simulink model "torqueBalancing2012b"  (Simulink 8.1)
settings: Solver=FixedStepDiscrete  StartTime=0.0  StopTime="CONFIG.SIMULATION_TIME "  FixedStep=CONFIG.Ts  RelTol=1e-3
InitFcn:
  | cd(fileparts(which(bdroot)));
  | initTorqueBalancing;
values from neighbouring files (symbols this model uses):
  WBT_modelName = 'matlabTorqueBalancing'    [InitMeasure.m]    (also in initTorqueBalancing.m)
undefined symbols (not defined in the file or in its folder): bVectorConstraintsFeet, bVectorConstraintsLegs, CONFIG, ConstraintsMatrixFeet, ConstraintsMatrixLegs, DiscIntNeverNeededParam, gain, references, reg, ROBOT_DOF, ROBOT_DOF_FOR_SIMULINK, sat, SM, sm, WBT_robotName
libraries: WBToolboxLibrary x182, simulink x13
(part 2 of 4)

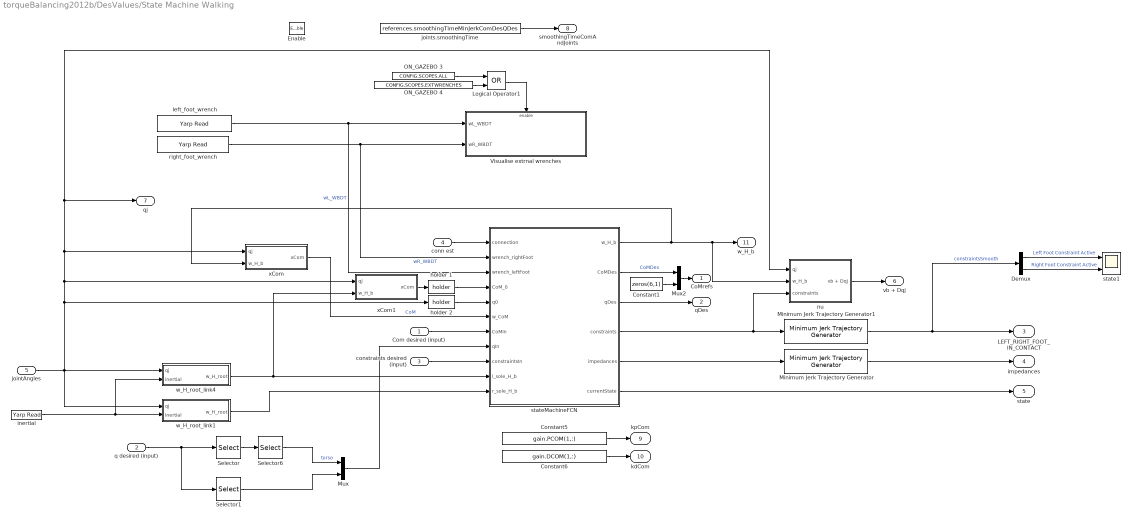
== system torqueBalancing2012b/DesValues/State Machine Walking ==
  Com desired (input) : Inport
  q desired (input) : Inport  Port=2
  constraints desired (input) : Inport  Port=3
  conn est : Inport  Port=4
  jointAngles : Inport  Port=5
  Enable : EnablePort
  Constant1 : Constant  Value=zeros(6,1)
  Constant5 : Constant  Value=gain.PCOM(1,:)
  Constant6 : Constant  Value=gain.DCOM(1,:)
  Demux : Demux  Outputs=2
  Logical Operator1 : Logic  Operator=OR  AllPortsSameDT=off  OutDataTypeStr=boolean
  Minimum Jerk Trajectory Generator : WBToolboxLibrary/Utilities/Minimum Jerk Trajectory Generator  externalSettlingTime=off  settlingTime=gain.SmoothingTimeImp  sampleTime=CONFIG.Ts  resetOnSettlingTime=off  firstDerivatives=off  secondDerivatives=off  explicitInitialValue=off
  Minimum Jerk Trajectory Generator1 : WBToolboxLibrary/Utilities/Minimum Jerk Trajectory Generator  externalSettlingTime=off  settlingTime=CONFIG.smoothingTimeTranDynamics  sampleTime=CONFIG.Ts  resetOnSettlingTime=off  firstDerivatives=off  secondDerivatives=off  explicitInitialValue=off
  Mux : Mux  Inputs=2
  Mux2 : Mux  Inputs=2
  ON_GAZEBO 3 : Constant  Value=CONFIG.SCOPES.ALL
  ON_GAZEBO 4 : Constant  Value=CONFIG.SCOPES.EXTWRENCHES
  Selector : Selector  InputPortWidth=ROBOT_DOF  IndexOptions=Index vector (dialog)  Indices=[1:3]  OutputSizes=1
  Selector1 : Selector  InputPortWidth=ROBOT_DOF  IndexOptions=Index vector (dialog)  Indices=[4:ROBOT_DOF]  OutputSizes=1
  Selector6 : Selector  InputPortWidth=3  IndexOptions=Index vector (dialog)  Indices=[3 2 1]  OutputSizes=1
  "Visualise extrnal wrenches  " : Subsystem
  holder 1 : WBToolboxLibrary/Utilities/holder 
  holder 2 : WBToolboxLibrary/Utilities/holder 
  inertial : WBToolboxLibrary/Utilities/Yarp Read  portName=PORTS.IMU  signalSize=12  blocking=off  timestamp=off  autoconnect=on  errorOnConnection=off
  joints.smoothingTime : Constant  Value=references.smoothingTimeMinJerkComDesQDes
  left_foot_wrench : WBToolboxLibrary/Utilities/Yarp Read  portName=PORTS.WBDT_LEFTLEG_EE  signalSize=6  blocking=off  timestamp=off  autoconnect=on  errorOnConnection=off
  nu : Subsystem
  right_foot_wrench : WBToolboxLibrary/Utilities/Yarp Read  portName=PORTS.WBDT_RIGHTLEG_EE  signalSize=6  blocking=off  timestamp=off  autoconnect=on  errorOnConnection=off
  state1 : Scope  NumInputPorts=2
      settings: YMin=-0.14635~-0.14635  YMax=1.12737~1.12737  SaveName=ScopeData2
  stateMachineFCN : MATLAB Function  Priority=-1  TreatAsAtomicUnit=on
  w_H_root_link1 : Subsystem  mask{link_name='r_sole'}
      mask prompts: link_name "link name"
      mask help:
      | This block evaluates the homogeneous transformation between the world and the root link, i.e. ^wH_b. It assumes that the link specified by the variable 'link_name' has a constant position
      | w.r.t. an inertial frame, but it can rotate arbitrarily. This rotation is retrived from the IMU sensor.
      mask Display:
      | str = strrep(link_name, '_','\_');
      | port_label('output',1,['{}^{',str '}H_{root}'],'texmode','on')
      | clear str;
      | 
      | port_label('input',1,'q_j','texmode','on')
      | 
      | port_label('input',2,'inertial','texmode','on')
  w_H_root_link4 : Subsystem  mask{link_name='l_sole'}
      mask prompts: link_name "link name"
      mask help:
      | This block evaluates the homogeneous transformation between the world and the root link, i.e. ^wH_b. It assumes that the link specified by the variable 'link_name' has a constant position
      | w.r.t. an inertial frame, but it can rotate arbitrarily. This rotation is retrived from the IMU sensor.
      mask Display:
      | str = strrep(link_name, '_','\_');
      | port_label('output',1,['{}^{',str '}H_{root}'],'texmode','on')
      | clear str;
      | 
      | port_label('input',1,'q_j','texmode','on')
      | 
      | port_label('input',2,'inertial','texmode','on')
  xCom : Subsystem  Priority=-2
  xCom1 : Subsystem  Priority=-2
  CoMrefs : Outport
  qDes : Outport  Port=2
  LEFT_RIGHT_FOOT_IN_CONTACT : Outport  Port=3
  impedances : Outport  Port=4
  state : Outport  Port=5
  vb + Dqj : Outport  Port=6
  qj : Outport  Port=7
  smoothingTimeComAndJoints : Outport  Port=8
  kpCom : Outport  Port=9
  kdCom : Outport  Port=10
  w_H_b : Outport  Port=11
  wires:
  xCom/1(xCom) -> stateMachineFCN/6(w_CoM)  "CoM"
  holder 2/1 -> stateMachineFCN/5(q0)
  stateMachineFCN/3(qDes) -> qDes/1
  stateMachineFCN/2(CoMDes) -> Mux2/1  "CoMDes"
  Mux2/1 -> CoMrefs/1
  Constant1/1 -> Mux2/2
  stateMachineFCN/5(impedances) -> Minimum Jerk Trajectory Generator/1
  stateMachineFCN/6(currentState) -> state/1
  Minimum Jerk Trajectory Generator1/1 -> Demux/1, LEFT_RIGHT_FOOT_IN_CONTACT/1  "constraintsSmooth"
  stateMachineFCN/4(constraints) -> nu/3("constraints "), Minimum Jerk Trajectory Generator1/1
  Demux/1 -> state1/1  "Left Foot Constraint Active"
  Demux/2 -> state1/2  "Right Foot Constraint Active"
  stateMachineFCN/1(w_H_b) -> xCom/2(w_H_b), nu/2(w_H_b), w_H_b/1
  nu/1(vb + Dqj) -> vb + Dqj/1
  Minimum Jerk Trajectory Generator/1 -> impedances/1
  w_H_root_link4/1(w_H_root) -> xCom1/2(w_H_b), stateMachineFCN/10(l_sole_H_b)
  w_H_root_link1/1(w_H_root) -> stateMachineFCN/11(r_sole_H_b)
  jointAngles/1 -> w_H_root_link1/1(qj), w_H_root_link4/1(qj), xCom1/1(qj), qj/1, nu/1(qj), xCom/1(qj), holder 2/1
  inertial/1 -> w_H_root_link4/2(inertial), w_H_root_link1/2(inertial)
  Com desired (input)/1 -> stateMachineFCN/7(CoMIn)
  constraints desired (input)/1 -> stateMachineFCN/9(constraintsIn)
  holder 1/1 -> stateMachineFCN/4(CoM_0)
  xCom1/1(xCom) -> holder 1/1
  conn est/1 -> stateMachineFCN/1(connection)
  q desired (input)/1 -> Selector1/1, Selector/1
  Selector6/1 -> Mux/1  "torso"
  Selector/1 -> Selector6/1
  Selector1/1 -> Mux/2
  Mux/1 -> stateMachineFCN/8(qIn)
  joints.smoothingTime/1 -> smoothingTimeComAndJoints/1
  right_foot_wrench/1 -> stateMachineFCN/2(wrench_rightFoot), "Visualise extrnal wrenches  "/2(wR_WBDT)  "wR_WBDT"
  left_foot_wrench/1 -> "Visualise extrnal wrenches  "/1(wL_WBDT), stateMachineFCN/3(wrench_leftFoot)  "wL_WBDT"
  Logical Operator1/1 -> "Visualise extrnal wrenches  "/Enable
  ON_GAZEBO 3/1 -> Logical Operator1/1
  ON_GAZEBO 4/1 -> Logical Operator1/2
  Constant5/1 -> kpCom/1
  Constant6/1 -> kdCom/1

== system torqueBalancing2012b/DesValues/Subsystem ==
  conn status 1 : Inport
  conn status 2 : Inport  Port=2
  conn status 3 : Inport  Port=3
  Compare To Zero3 : simulink/Logic and Bit Operations/Compare To Zero  relop=>  OutDataTypeStr=boolean
  Compare To Zero4 : simulink/Logic and Bit Operations/Compare To Zero  relop=>  OutDataTypeStr=boolean
  Compare To Zero5 : simulink/Logic and Bit Operations/Compare To Zero  relop=>  OutDataTypeStr=boolean
  Logical Operator : Logic  Inputs=3  AllPortsSameDT=off  OutDataTypeStr=boolean
  connection check : Outport
  wires:
  Logical Operator/1 -> connection check/1
  Compare To Zero4/1 -> Logical Operator/3
  conn status 1/1 -> Compare To Zero3/1
  Compare To Zero3/1 -> Logical Operator/1
  conn status 3/1 -> Compare To Zero4/1
  Compare To Zero5/1 -> Logical Operator/2
  conn status 2/1 -> Compare To Zero5/1

== system torqueBalancing2012b/Dump and visualize/ZMPs ==
  fDesQP : Inport
  Demux1 : Demux  Outputs=3
  Demux2 : Demux  Outputs=3
  Divide{4..7} (4 alike) : Product  Inputs=*/
  Gain3 : Gain  Gain=-1
  Gain4 : Gain  Gain=-1
  Mux : Mux  Inputs=2
  Mux1 : Mux  Inputs=2
  fz taux tauy Left : Selector  InputPortWidth=12  IndexOptions=Index vector (dialog)  Indices=[3 4 5]  OutputSizes=1
  fz taux tauy Right : Selector  InputPortWidth=12  IndexOptions=Index vector (dialog)  Indices=[9 10 11]  OutputSizes=1
  ZMP_LeftFoot : Outport
  ZMP_RightFoot : Outport  Port=2
  wires:
  fz taux tauy Left/1 -> Demux1/1
  Demux1/1 -> Divide4/2, Divide5/2
  Divide7/1 -> Gain4/1
  Divide4/1 -> Mux/2
  Divide5/1 -> Gain3/1
  fz taux tauy Right/1 -> Demux2/1
  Demux2/1 -> Divide6/2, Divide7/2
  fDesQP/1 -> fz taux tauy Left/1, fz taux tauy Right/1
  Gain3/1 -> Mux/1
  Mux/1 -> ZMP_LeftFoot/1
  Divide6/1 -> Mux1/2
  Gain4/1 -> Mux1/1
  Mux1/1 -> ZMP_RightFoot/1
  Demux1/2 -> Divide4/1  "tauxL"
  Demux1/3 -> Divide5/1  "tauyL"
  Demux2/2 -> Divide6/1  "tauxR"
  Demux2/3 -> Divide7/1  "tauyR"

== system torqueBalancing2012b/Dump and visualize/plotNorms ==
  qTile_LeftLeg : Inport
  qTile_RightLeg : Inport  Port=2
  state : Inport  Port=3
  Constant : Constant  Value=sm.joints.thresholdInContact
  Constant2 : Constant  Value=sm.joints.thresholdNotInContact
  Mux : Mux  Inputs=3
  Mux1 : Mux  Inputs=3
  norm : MATLAB Function  TreatAsAtomicUnit=on
  norm(qTilde) : Scope  NumInputPorts=3
      settings: ShowLegends=on  YMin=-6.25~-6.25~-6.25  YMax=56.25~56.25~56.25
  norm1 : MATLAB Function  TreatAsAtomicUnit=on
  wires:
  Constant/1 -> Mux1/2, Mux/2  "thresholdInContact"
  qTile_LeftLeg/1 -> norm1/1(u)
  qTile_RightLeg/1 -> norm/1(u)
  norm/1(normU) -> Mux1/1  "norm(qTilde_RightL)"
  norm1/1(normU) -> Mux/1  "norm(qTilde_LeftL)"
  Mux/1 -> norm(qTilde)/1
  Mux1/1 -> norm(qTilde)/2
  Constant2/1 -> Mux1/3, Mux/3  "thresholdNotInContact"
  state/1 -> norm(qTilde)/3

== system torqueBalancing2012b/controller_QP/Arm External Forces ==
  w_H_b : Inport
  qj : Inport  Port=2
  r_sole1 : WBToolboxLibrary/wholeBodyModel/Kinematics/Forward Kinematics  frameName='r_hand_dh_frame'  robotName=WBT_robotName  localName=WBT_modelName  wbiFile=WBT_wbiFilename  wbiList=WBT_wbiList
  r_sole2 : WBToolboxLibrary/wholeBodyModel/Kinematics/Forward Kinematics  frameName='l_hand_dh_frame'  robotName=WBT_robotName  localName=WBT_modelName  wbiFile=WBT_wbiFilename  wbiList=WBT_wbiList
  w_H_LArm : Outport
  w_H_RArm : Outport  Port=2
  wires:
  qj/1 -> r_sole2/2, r_sole1/2
  r_sole1/1 -> w_H_RArm/1
  w_H_b/1 -> r_sole2/1, r_sole1/1
  r_sole2/1 -> w_H_LArm/1

== system torqueBalancing2012b/controller_QP/Constraints ==
  legsInContact : Inport
  Constant : Constant  Value=ConstraintsMatrixFeet
  Constant1 : Constant  Value=bVectorConstraintsLegs
  Constant2 : Constant  Value=ConstraintsMatrixLegs
  Constant3 : Constant  Value=bVectorConstraintsFeet
  Switch1 : Switch  Criteria=u2 > Threshold
  Switch2 : Switch  Criteria=u2 > Threshold
  ConstraintsMatrix : Outport
  bVectorConstraints : Outport  Port=2
  wires:
  Constant2/1 -> Switch1/1
  Constant1/1 -> Switch2/1
  legsInContact/1 -> Switch2/2, Switch1/2
  Constant/1 -> ConstraintsMatrix/1, Switch1/3
  Constant3/1 -> bVectorConstraints/1, Switch2/3

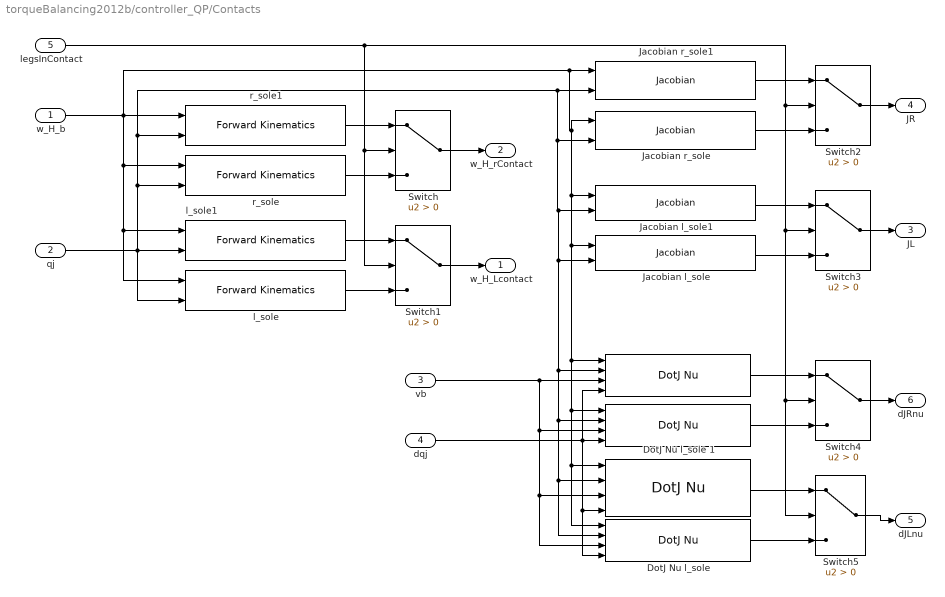
== system torqueBalancing2012b/controller_QP/Contacts ==
  w_H_b : Inport
  qj : Inport  Port=2
  vb : Inport  Port=3
  dqj : Inport  Port=4
  legsInContact : Inport  Port=5
  " " : WBToolboxLibrary/wholeBodyModel/Jacobians/DotJ Nu  frameName='r_upper_leg_contact'  robotName=WBT_robotName  localName=WBT_modelName  wbiFile=WBT_wbiFilename  wbiList=WBT_wbiList
  "    " : WBToolboxLibrary/wholeBodyModel/Jacobians/DotJ Nu  frameName='r_sole'  robotName=WBT_robotName  localName=WBT_modelName  wbiFile=WBT_wbiFilename  wbiList=WBT_wbiList
  "DotJ Nu l_sole " : WBToolboxLibrary/wholeBodyModel/Jacobians/DotJ Nu  frameName='l_sole'  robotName=WBT_robotName  localName=WBT_modelName  wbiFile=WBT_wbiFilename  wbiList=WBT_wbiList
  DotJ Nu l_sole 1 : WBToolboxLibrary/wholeBodyModel/Jacobians/DotJ Nu  frameName='l_upper_leg_contact'  robotName=WBT_robotName  localName=WBT_modelName  wbiFile=WBT_wbiFilename  wbiList=WBT_wbiList
  Jacobian l_sole : WBToolboxLibrary/wholeBodyModel/Jacobians/Jacobian  frameName='l_sole'  robotName=WBT_robotName  localName=WBT_modelName  wbiFile=WBT_wbiFilename  wbiList=WBT_wbiList
  Jacobian l_sole1 : WBToolboxLibrary/wholeBodyModel/Jacobians/Jacobian  frameName='l_upper_leg_contact'  robotName=WBT_robotName  localName=WBT_modelName  wbiFile=WBT_wbiFilename  wbiList=WBT_wbiList
  Jacobian r_sole : WBToolboxLibrary/wholeBodyModel/Jacobians/Jacobian  frameName='r_sole'  robotName=WBT_robotName  localName=WBT_modelName  wbiFile=WBT_wbiFilename  wbiList=WBT_wbiList
  Jacobian r_sole1 : WBToolboxLibrary/wholeBodyModel/Jacobians/Jacobian  frameName='r_upper_leg_contact'  robotName=WBT_robotName  localName=WBT_modelName  wbiFile=WBT_wbiFilename  wbiList=WBT_wbiList
  Switch{,1..5} (6 alike) : Switch  Criteria=u2 > Threshold
  l_sole : WBToolboxLibrary/wholeBodyModel/Kinematics/Forward Kinematics  frameName='l_sole'  robotName=WBT_robotName  localName=WBT_modelName  wbiFile=WBT_wbiFilename  wbiList=WBT_wbiList
  l_sole1 : WBToolboxLibrary/wholeBodyModel/Kinematics/Forward Kinematics  frameName='l_upper_leg_contact'  robotName=WBT_robotName  localName=WBT_modelName  wbiFile=WBT_wbiFilename  wbiList=WBT_wbiList
  r_sole : WBToolboxLibrary/wholeBodyModel/Kinematics/Forward Kinematics  frameName='r_sole'  robotName=WBT_robotName  localName=WBT_modelName  wbiFile=WBT_wbiFilename  wbiList=WBT_wbiList
  r_sole1 : WBToolboxLibrary/wholeBodyModel/Kinematics/Forward Kinematics  frameName='r_upper_leg_contact'  robotName=WBT_robotName  localName=WBT_modelName  wbiFile=WBT_wbiFilename  wbiList=WBT_wbiList
  w_H_Lcontact : Outport
  w_H_rContact : Outport  Port=2
  JL : Outport  Port=3
  JR : Outport  Port=4
  dJLnu : Outport  Port=5
  dJRnu : Outport  Port=6
  wires:
  r_sole1/1 -> Switch/1
  r_sole/1 -> Switch/3
  l_sole1/1 -> Switch1/1
  l_sole/1 -> Switch1/3
  w_H_b/1 -> Jacobian l_sole1/1, "DotJ Nu l_sole "/1, DotJ Nu l_sole 1/1, "    "/1, " "/1, Jacobian l_sole/1, Jacobian r_sole/1, Jacobian r_sole1/1, r_sole1/1, l_sole/1, l_sole1/1, r_sole/1
  Jacobian r_sole1/1 -> Switch2/1
  legsInContact/1 -> Switch1/2, Switch/2, Switch5/2, Switch4/2, Switch3/2, Switch2/2
  Jacobian r_sole/1 -> Switch2/3
  Jacobian l_sole1/1 -> Switch3/1
  qj/1 -> l_sole/2, "DotJ Nu l_sole "/2, DotJ Nu l_sole 1/2, "    "/2, " "/2, Jacobian l_sole/2, Jacobian l_sole1/2, Jacobian r_sole/2, Jacobian r_sole1/2, r_sole1/2, r_sole/2, l_sole1/2
  vb/1 -> "DotJ Nu l_sole "/3, DotJ Nu l_sole 1/3, "    "/3, " "/3
  dqj/1 -> "DotJ Nu l_sole "/4, DotJ Nu l_sole 1/4, " "/4, "    "/4
  " "/1 -> Switch4/1
  "    "/1 -> Switch4/3
  DotJ Nu l_sole 1/1 -> Switch5/1
  "DotJ Nu l_sole "/1 -> Switch5/3
  Jacobian l_sole/1 -> Switch3/3
  Switch/1 -> w_H_rContact/1
  Switch1/1 -> w_H_Lcontact/1
  Switch3/1 -> JL/1
  Switch2/1 -> JR/1
  Switch4/1 -> dJRnu/1
  Switch5/1 -> dJLnu/1

== system torqueBalancing2012b/controller_QP/QP ==
  LEFT_RIGHT_FOOT_IN_CONTACT : Inport
  HessianMatrixQP1Foot : Inport  Port=2
  gradientQP1Foot : Inport  Port=3
  ConstraintsMatrixQP1Foot : Inport  Port=4
  bVectorConstraintsQP1Foot : Inport  Port=5
  HessianMatrixQP2FeetOrLegs : Inport  Port=6
  gradientQP2FeetOrLegs : Inport  Port=7
  ConstraintsMatrixQP2FeetOrLegs : Inport  Port=8
  bVectorConstraintsQp2FeetOrLegs : Inport  Port=9
  state : Inport  Port=10
  Constant1 : Constant  Value=CONFIG.USE_QP_SOLVER
  Level-2 MATLAB S-Function : M-S-Function  FunctionName=QpBalancing
  Logical Operator1 : Logic  Operator=OR  AllPortsSameDT=off  OutDataTypeStr=boolean
  ON_GAZEBO 3 : Constant  Value=CONFIG.SCOPES.ALL
  ON_GAZEBO 4 : Constant  Value=CONFIG.SCOPES.QP
  QP two feet fails : Assertion  Commented=on
  Visualize eventual QP failures : Subsystem
  f0OneFoot : Outport
  f0TwoFeet : Outport  Port=2
  wires:
  Level-2 MATLAB S-Function/1 -> f0TwoFeet/1
  Level-2 MATLAB S-Function/2 -> Visualize eventual QP failures/1(exitFlagQP), QP two feet fails/1  "Exit flag QP two feet"
  HessianMatrixQP1Foot/1 -> Level-2 MATLAB S-Function/7
  gradientQP1Foot/1 -> Level-2 MATLAB S-Function/8
  ConstraintsMatrixQP1Foot/1 -> Level-2 MATLAB S-Function/9
  bVectorConstraintsQP1Foot/1 -> Level-2 MATLAB S-Function/10
  Level-2 MATLAB S-Function/3 -> f0OneFoot/1
  Logical Operator1/1 -> Visualize eventual QP failures/Enable
  state/1 -> Visualize eventual QP failures/2(state)
  LEFT_RIGHT_FOOT_IN_CONTACT/1 -> Level-2 MATLAB S-Function/1
  HessianMatrixQP2FeetOrLegs/1 -> Level-2 MATLAB S-Function/2
  gradientQP2FeetOrLegs/1 -> Level-2 MATLAB S-Function/3
  ConstraintsMatrixQP2FeetOrLegs/1 -> Level-2 MATLAB S-Function/4
  bVectorConstraintsQp2FeetOrLegs/1 -> Level-2 MATLAB S-Function/5
  Constant1/1 -> Level-2 MATLAB S-Function/6
  ON_GAZEBO 3/1 -> Logical Operator1/1
  ON_GAZEBO 4/1 -> Logical Operator1/2

== system torqueBalancing2012b/controller_QP/integralOf Hw1 ==
  qjDes : Inport
  qj : Inport  Port=2
  constraints : Inport  Port=3
  legsInContact : Inport  Port=4
  " " : WBToolboxLibrary/wholeBodyModel/Jacobians/Jacobian  frameName='l_upper_leg_contact'  robotName=WBT_robotName  localName=WBT_modelName  wbiFile=WBT_wbiFilename  wbiList=WBT_wbiList
  "  " : WBToolboxLibrary/wholeBodyModel/Jacobians/Jacobian  frameName='r_upper_leg_contact'  robotName=WBT_robotName  localName=WBT_modelName  wbiFile=WBT_wbiFilename  wbiList=WBT_wbiList
  "   " : WBToolboxLibrary/wholeBodyModel/Jacobians/Jacobian  frameName='r_sole'  robotName=WBT_robotName  localName=WBT_modelName  wbiFile=WBT_wbiFilename  wbiList=WBT_wbiList
  "       " : WBToolboxLibrary/wholeBodyModel/Jacobians/Jacobian  frameName='l_sole'  robotName=WBT_robotName  localName=WBT_modelName  wbiFile=WBT_wbiFilename  wbiList=WBT_wbiList
  Centroidal Momentum : WBToolboxLibrary/wholeBodyModel/Dynamics/Centroidal Momentum  robotName=WBT_robotName  localName=WBT_modelName  wbiFile=WBT_wbiFilename  wbiList=WBT_wbiList
  MATLAB Function : MATLAB Function  TreatAsAtomicUnit=on
  Selector : Selector  InputPortWidth=6  IndexOptions=Index vector (dialog)  Indices=[4 5 6]  OutputSizes=1
  Sum : Sum  Inputs=|-+
  Switch : Switch  Criteria=u2 > Threshold
  Switch1 : Switch  Criteria=u2 > Threshold
  Switch2 : Switch  Criteria=u2 > Threshold
  inertial : WBToolboxLibrary/Utilities/Yarp Read  portName=PORTS.IMU  signalSize=12  blocking=off  timestamp=off  autoconnect=on  errorOnConnection=on
  inertial1 : WBToolboxLibrary/Utilities/Yarp Read  portName=PORTS.IMU  signalSize=12  blocking=off  timestamp=off  autoconnect=on  errorOnConnection=on
  w_H_root_link1 : Subsystem  mask{link_name='l_upper_leg_contact'}
      mask prompts: link_name "link name"
      mask help:
      | This block evaluates the homogeneous transformation between the world and the root link, i.e. ^wH_b. It assumes that the link specified by the variable 'link_name' has a constant position
      | w.r.t. an inertial frame, but it can rotate arbitrarily. This rotation is retrived from the IMU sensor.
      mask Display:
      | str = strrep(link_name, '_','\_');
      | port_label('output',1,['{}^{',str '}H_{root}'],'texmode','on')
      | clear str;
      | 
      | port_label('input',1,'q_j','texmode','on')
      | 
      | port_label('input',2,'inertial','texmode','on')
  w_H_root_link4 : Subsystem  mask{link_name='l_sole'}
      mask prompts: link_name "link name"
      mask help:
      | This block evaluates the homogeneous transformation between the world and the root link, i.e. ^wH_b. It assumes that the link specified by the variable 'link_name' has a constant position
      | w.r.t. an inertial frame, but it can rotate arbitrarily. This rotation is retrived from the IMU sensor.
      mask Display:
      | str = strrep(link_name, '_','\_');
      | port_label('output',1,['{}^{',str '}H_{root}'],'texmode','on')
      | clear str;
      | 
      | port_label('input',1,'q_j','texmode','on')
      | 
      | port_label('input',2,'inertial','texmode','on')
  intHw : Outport
  wires:
  qj/1 -> Sum/2
  Sum/1 -> Centroidal Momentum/4, MATLAB Function/1(qjErr)
  Centroidal Momentum/1 -> Selector/1
  Selector/1 -> intHw/1
  constraints/1 -> MATLAB Function/4(activeFeetConstraints)
  inertial/1 -> w_H_root_link4/2(inertial)
  qjDes/1 -> "   "/2, Sum/1, "  "/2, "       "/2, Centroidal Momentum/2, " "/2, w_H_root_link4/1(qj), w_H_root_link1/1(qj)
  inertial1/1 -> w_H_root_link1/2(inertial)
  w_H_root_link1/1(w_H_root) -> Switch/1
  legsInContact/1 -> Switch2/2, Switch1/2, Switch/2
  " "/1 -> Switch1/1
  "  "/1 -> Switch2/1
  "       "/1 -> Switch1/3
  "   "/1 -> Switch2/3
  MATLAB Function/1(vbEquivalent) -> Centroidal Momentum/3
  Switch2/1 -> MATLAB Function/3(JR)
  Switch1/1 -> MATLAB Function/2(JL)
  w_H_root_link4/1(w_H_root) -> Switch/3
  Switch/1 -> "       "/1, "  "/1, "   "/1, " "/1, Centroidal Momentum/1

== system torqueBalancing2012b/controller_QP/xCom ==
  w_H_b : Inport
  qj : Inport  Port=2
  "CoM6D ->  CoMXYZ2" : Selector  NumberOfDimensions=2  InputPortWidth=7  IndexOptions=Index vector (dialog),Index vector (dialog)  Indices=[1 2 3],[4]  OutputSizes=1,1
  com : WBToolboxLibrary/wholeBodyModel/Kinematics/Forward Kinematics  frameName='com'  robotName=WBT_robotName  localName=WBT_modelName  wbiFile=WBT_wbiFilename  wbiList=WBT_wbiList
  xCom : Outport
  wires:
  qj/1 -> com/2
  "CoM6D ->  CoMXYZ2"/1 -> xCom/1
  com/1 -> "CoM6D ->  CoMXYZ2"/1
  w_H_b/1 -> com/1

== system torqueBalancing2012b/controller_QP/xCom1 ==
  w_H_b : Inport
  qj : Inport  Port=2
  "CoM6D ->  CoMXYZ2" : Selector  NumberOfDimensions=2  InputPortWidth=7  IndexOptions=Index vector (dialog),Index vector (dialog)  Indices=[1 2 3],[4]  OutputSizes=1,1
  com : WBToolboxLibrary/wholeBodyModel/Kinematics/Forward Kinematics  frameName='com'  robotName=WBT_robotName  localName=WBT_modelName  wbiFile=WBT_wbiFilename  wbiList=WBT_wbiList
  xCom : Outport
  wires:
  qj/1 -> com/2
  "CoM6D ->  CoMXYZ2"/1 -> xCom/1
  com/1 -> "CoM6D ->  CoMXYZ2"/1
  w_H_b/1 -> com/1

== system torqueBalancing2012b/record results/ZMPs ==
  fDesQP : Inport
  Lcontact : Inport  Port=2
  Rcontact : Inport  Port=3
  Demux1 : Demux  Outputs=3
  Demux2 : Demux  Outputs=3
  Divide{4..7} (4 alike) : Product  Inputs=*/
  Gain3 : Gain  Gain=-1
  Gain4 : Gain  Gain=-1
  MATLAB Function : MATLAB Function  TreatAsAtomicUnit=on
  Vector Concatenate : Concatenate  Mode=Multidimensional array
  Vector Concatenate1 : Concatenate  Mode=Multidimensional array
  fz taux tauy Left : Selector  InputPortWidth=12  IndexOptions=Index vector (dialog)  Indices=[3 4 5]  OutputSizes=1
  fz taux tauy Right : Selector  InputPortWidth=12  IndexOptions=Index vector (dialog)  Indices=[9 10 11]  OutputSizes=1
  zmp : Outport
  wires:
  fz taux tauy Left/1 -> Demux1/1
  Demux1/1 -> MATLAB Function/1(fz_left), Divide4/2, Divide5/2
  Divide7/1 -> Gain4/1
  Divide4/1 -> Vector Concatenate/2
  Divide5/1 -> Gain3/1
  fz taux tauy Right/1 -> Demux2/1
  Demux2/1 -> MATLAB Function/2(fz_right), Divide6/2, Divide7/2
  fDesQP/1 -> fz taux tauy Left/1, fz taux tauy Right/1
  Gain3/1 -> Vector Concatenate/1
  Vector Concatenate/1 -> MATLAB Function/3(Lcop)
  Divide6/1 -> Vector Concatenate1/2
  Gain4/1 -> Vector Concatenate1/1
  Vector Concatenate1/1 -> MATLAB Function/4(Rcop)
  Demux1/2 -> Divide4/1  "tauxL"
  Demux1/3 -> Divide5/1  "tauyL"
  Demux2/2 -> Divide6/1  "tauxR"
  Demux2/3 -> Divide7/1  "tauyR"
  Lcontact/1 -> MATLAB Function/5(Lcontact)
  Rcontact/1 -> MATLAB Function/6(Rcontact)
  MATLAB Function/1(zmp) -> zmp/1

== system torqueBalancing2012b/synchronizer/GAZEBO_SYNCHRONIZER ==
  Enable : EnablePort
  Simulator Synchronizer : WBToolboxLibrary/Utilities/Simulator Synchronizer  period=CONFIG.Ts  serverPortName='/clock/rpc'  clientPortName='/WBT_synchronizer/rpc:o'

== system torqueBalancing2012b/synchronizer/REAL_TIME_SYNC ==
  Enable : EnablePort
  Real Time Synchronizer : WBToolboxLibrary/Utilities/Real Time Synchronizer  period=CONFIG.Ts

== system torqueBalancing2012b/DesValues/Internal coordinator/nu ==
  qj : Inport
  w_H_b : Inport  Port=2
  "constraints " : Inport  Port=3
  Get Estimate : WBToolboxLibrary/wholeBodyStates/Get Estimate  estimateType=Joints Velocity  robotName=WBT_robotName  localName=WBT_modelName  wbiFile=WBT_wbiFilename  wbiList=WBT_wbiList
  Jacobian l_sole : WBToolboxLibrary/wholeBodyModel/Jacobians/Jacobian  frameName='l_sole'  robotName=WBT_robotName  localName=WBT_modelName  wbiFile=WBT_wbiFilename  wbiList=WBT_wbiList
  Jacobian r_sole : WBToolboxLibrary/wholeBodyModel/Jacobians/Jacobian  frameName='r_sole'  robotName=WBT_robotName  localName=WBT_modelName  wbiFile=WBT_wbiFilename  wbiList=WBT_wbiList
  MATLAB Function : MATLAB Function  TreatAsAtomicUnit=on
  Mux : Mux  Inputs=2
  vb + Dqj : Outport
  wires:
  Get Estimate/1 -> MATLAB Function/4(qD), Mux/2
  Mux/1 -> vb + Dqj/1
  Jacobian r_sole/1 -> MATLAB Function/2(JcRightFoot)
  "constraints "/1 -> MATLAB Function/3(activeFeetConstraints)
  MATLAB Function/1(y) -> Mux/1
  Jacobian l_sole/1 -> MATLAB Function/1(JcLeftFoot)
  qj/1 -> Jacobian l_sole/2, Jacobian r_sole/2
  w_H_b/1 -> Jacobian l_sole/1, Jacobian r_sole/1

== system torqueBalancing2012b/DesValues/Internal coordinator/refGen ==
  Enable : EnablePort
  Clock2 : Clock
  Display : Display
  Display1 : Display
  Display2 : Display
  XcomDes : FromWorkspace  VariableName=ts_xCoMDes  SampleTime=0
  "com reference " : MATLAB Function  TreatAsAtomicUnit=on
  dXcomDes : FromWorkspace  VariableName=ts_dxCoMDes  SampleTime=0
  ddXcomDes : FromWorkspace  VariableName=ts_ddxCoMDes  SampleTime=0
  holder 1 : WBToolboxLibrary/Utilities/holder 
  "joint reference " : MATLAB Function  TreatAsAtomicUnit=on
  parameters1 : Constant  Value=CONFIG.JOINTS
  parameters2 : Constant  Value=CONFIG.TIME_CONTROLLER_SWITCH
  parameters3 : Constant  Value=CONFIG.JOINTSITING
  parameters4 : Constant  Value=CONFIG.FIXEDCOMBENCH
  qDes : Outport
  CoMrefs : Outport  Port=2
  wires:
  Clock2/1 -> "joint reference "/1(t), "com reference "/1(t)
  "com reference "/1(Comrefs) -> CoMrefs/1
  XcomDes/1 -> Display1/1, "com reference "/4(xCoMDes), holder 1/1
  holder 1/1 -> Display/1, "com reference "/3(first_xCom)
  dXcomDes/1 -> "com reference "/5(dxCoMDes)
  ddXcomDes/1 -> "com reference "/6(ddxCoMDes)
  "joint reference "/1(qdes) -> qDes/1
  parameters1/1 -> "joint reference "/4(final_joint)
  parameters3/1 -> "joint reference "/3(sitting_joint)
  parameters2/1 -> "joint reference "/2(t_switch), "com reference "/2(t_switch)
  parameters4/1 -> Display2/1, "com reference "/7(fixedComBench)

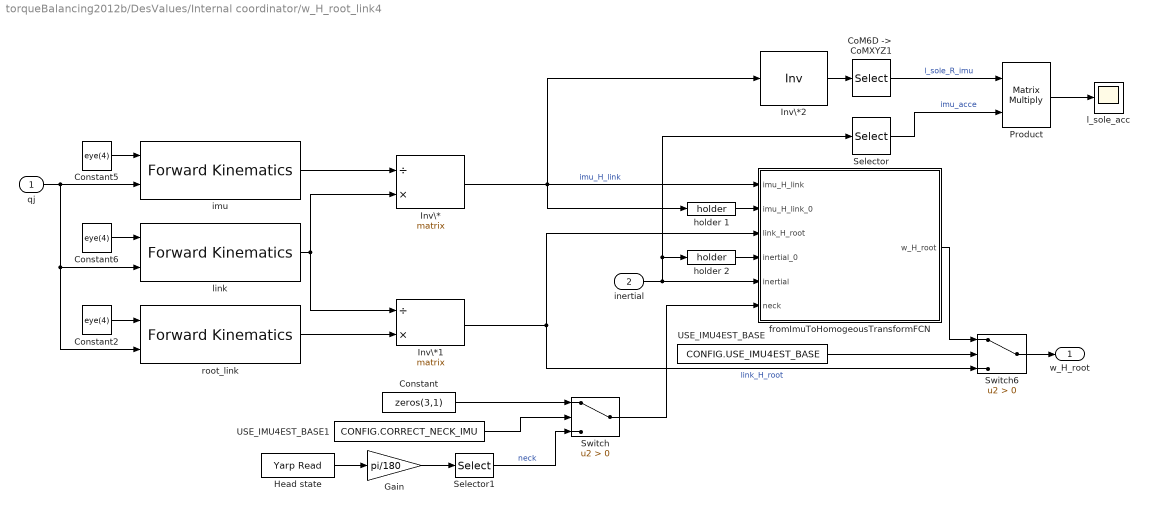
== system torqueBalancing2012b/DesValues/Internal coordinator/w_H_root_link4 ==
  qj : Inport
  inertial : Inport  Port=2
  "CoM6D ->  CoMXYZ1" : Selector  NumberOfDimensions=2  InputPortWidth=7  IndexOptions=Index vector (dialog),Index vector (dialog)  Indices=[1 2 3],[1 2 3]  OutputSizes=1,1
  Constant : Constant  Value=zeros(3,1)
  Constant2 : Constant  Value=eye(4)
  Constant5 : Constant  Value=eye(4)
  Constant6 : Constant  Value=eye(4)
  Gain : Gain  Gain=pi/180
  Head state : WBToolboxLibrary/Utilities/Yarp Read  portName=[WBT_robotName, '/head/state:o']  signalSize=6  blocking=off  timestamp=off  autoconnect=on  errorOnConnection=off
  Inv\* : Product  Inputs=/*  Multiplication=Matrix(*)
  Inv\*1 : Product  Inputs=/*  Multiplication=Matrix(*)
  Inv\*2 : Product  Inputs=/  Multiplication=Matrix(*)
  Product : Product  Multiplication=Matrix(*)
  Selector : Selector  InputPortWidth=12  IndexOptions=Index vector (dialog)  Indices=[4 5 6 ]  OutputSizes=1
  Selector1 : Selector  InputPortWidth=6  IndexOptions=Index vector (dialog)  Indices=[1:3]  OutputSizes=1
  Switch : Switch  Criteria=u2 > Threshold
  Switch6 : Switch  Criteria=u2 > Threshold
  USE_IMU4EST_BASE : Constant  Value=CONFIG.USE_IMU4EST_BASE
  USE_IMU4EST_BASE1 : Constant  Value=CONFIG.CORRECT_NECK_IMU
  fromImuToHomogeousTransformFCN : MATLAB Function  TreatAsAtomicUnit=on
  holder 1 : WBToolboxLibrary/Utilities/holder 
  holder 2 : WBToolboxLibrary/Utilities/holder 
  imu : WBToolboxLibrary/wholeBodyModel/Kinematics/Forward Kinematics  frameName='imu_frame'  robotName=WBT_robotName  localName=WBT_modelName  wbiFile=WBT_wbiFilename  wbiList=WBT_wbiList
  l_sole_acc : Scope
      settings: ShowLegends=on  TimeRange=60  YMin=-4.47309  YMax=14.2668
  link : WBToolboxLibrary/wholeBodyModel/Kinematics/Forward Kinematics  frameName=link_name  robotName=WBT_robotName  localName=WBT_modelName  wbiFile=WBT_wbiFilename  wbiList=WBT_wbiList
  root_link : WBToolboxLibrary/wholeBodyModel/Kinematics/Forward Kinematics  frameName='root_link'  robotName=WBT_robotName  localName=WBT_modelName  wbiFile=WBT_wbiFilename  wbiList=WBT_wbiList
  w_H_root : Outport
  wires:
  Constant5/1 -> imu/1
  Inv\*/1 -> Inv\*2/1, holder 1/1, fromImuToHomogeousTransformFCN/1(imu_H_link)  "imu_H_link"
  imu/1 -> Inv\*/1
  Constant6/1 -> link/1
  Inv\*1/1 -> Switch6/3, fromImuToHomogeousTransformFCN/3(link_H_root)  "link_H_root"
  link/1 -> Inv\*/2, Inv\*1/1
  inertial/1 -> Selector/1, holder 2/1, fromImuToHomogeousTransformFCN/5(inertial)
  Switch6/1 -> w_H_root/1
  USE_IMU4EST_BASE/1 -> Switch6/2
  fromImuToHomogeousTransformFCN/1(w_H_root) -> Switch6/1
  Constant2/1 -> root_link/1
  qj/1 -> root_link/2, link/2, imu/2
  root_link/1 -> Inv\*1/2
  holder 1/1 -> fromImuToHomogeousTransformFCN/2(imu_H_link_0)
  holder 2/1 -> fromImuToHomogeousTransformFCN/4(inertial_0)
  Inv\*2/1 -> "CoM6D ->  CoMXYZ1"/1
  "CoM6D ->  CoMXYZ1"/1 -> Product/1  "l_sole_R_imu"
  Selector/1 -> Product/2  "imu_acce"
  Product/1 -> l_sole_acc/1
  Head state/1 -> Gain/1
  Selector1/1 -> Switch/3  "neck"
  Constant/1 -> Switch/1
  USE_IMU4EST_BASE1/1 -> Switch/2
  Switch/1 -> fromImuToHomogeousTransformFCN/6(neck)
  Gain/1 -> Selector1/1

== system torqueBalancing2012b/DesValues/Internal coordinator/xCom ==
  w_H_b : Inport
  qj : Inport  Port=2
  "CoM6D ->  CoMXYZ2" : Selector  NumberOfDimensions=2  InputPortWidth=7  IndexOptions=Index vector (dialog),Index vector (dialog)  Indices=[1 2 3],[4]  OutputSizes=1,1
  com : WBToolboxLibrary/wholeBodyModel/Kinematics/Forward Kinematics  frameName='com'  robotName=WBT_robotName  localName=WBT_modelName  wbiFile=WBT_wbiFilename  wbiList=WBT_wbiList
  xCom : Outport
  wires:
  qj/1 -> com/2
  "CoM6D ->  CoMXYZ2"/1 -> xCom/1
  com/1 -> "CoM6D ->  CoMXYZ2"/1
  w_H_b/1 -> com/1

== system torqueBalancing2012b/DesValues/State Machine/Visualise extrnal wrenches   ==
  wL_WBDT : Inport
  wR_WBDT : Inport  Port=2
  Enable : EnablePort
  Constant : Constant  Value=sm.wrench.thresholdContactOn
  Constant2 : Constant  Value=sm.wrench.thresholdContactOff
  left foot ext wrench : Scope  NumInputPorts=3
      settings: YMin=81.68454~81.68454~81.68454  YMax=109.97631~109.97631~109.97631
  right foot ext wrench : Scope  NumInputPorts=3
      settings: ShowLegends=on  TimeRange=42.68  YMin=-65.30999~-65.30999~-65.30999  YMax=249.85279~249.85279~249.85279  SaveName=ScopeData2
  wires:
  Constant/1 -> left foot ext wrench/2, right foot ext wrench/2  "thresholdContactOn"
  wR_WBDT/1 -> right foot ext wrench/1  "wR_WBDT"
  wL_WBDT/1 -> left foot ext wrench/1  "wL_WBDT"
  Constant2/1 -> left foot ext wrench/3, right foot ext wrench/3  "thresholdContactOff"

== system torqueBalancing2012b/DesValues/State Machine/nu ==
  qj : Inport
  w_H_b : Inport  Port=2
  "constraints " : Inport  Port=3
  Get Estimate : WBToolboxLibrary/wholeBodyStates/Get Estimate  estimateType=Joints Velocity  robotName=WBT_robotName  localName=WBT_modelName  wbiFile=WBT_wbiFilename  wbiList=WBT_wbiList
  Jacobian l_sole : WBToolboxLibrary/wholeBodyModel/Jacobians/Jacobian  frameName='l_sole'  robotName=WBT_robotName  localName=WBT_modelName  wbiFile=WBT_wbiFilename  wbiList=WBT_wbiList
  Jacobian r_sole : WBToolboxLibrary/wholeBodyModel/Jacobians/Jacobian  frameName='r_sole'  robotName=WBT_robotName  localName=WBT_modelName  wbiFile=WBT_wbiFilename  wbiList=WBT_wbiList
  MATLAB Function : MATLAB Function  TreatAsAtomicUnit=on
  Mux : Mux  Inputs=2
  vb + Dqj : Outport
  wires:
  Get Estimate/1 -> MATLAB Function/4(qD), Mux/2
  Mux/1 -> vb + Dqj/1
  Jacobian r_sole/1 -> MATLAB Function/2(JcRightFoot)
  "constraints "/1 -> MATLAB Function/3(activeFeetConstraints)
  MATLAB Function/1(y) -> Mux/1
  Jacobian l_sole/1 -> MATLAB Function/1(JcLeftFoot)
  qj/1 -> Jacobian l_sole/2, Jacobian r_sole/2
  w_H_b/1 -> Jacobian r_sole/1, Jacobian l_sole/1

== system torqueBalancing2012b/DesValues/State Machine/visualise inertial ==
  jointAngles : Inport
  inertial : Inport  Port=2
  Enable : EnablePort
  Inv\* : Product  Inputs=/*  Multiplication=Matrix(*)
  Inv\*1 : Product  Inputs=/*  Multiplication=Matrix(*)
  Visualize hom transf2 : Subsystem
  Visualize hom transf4 : Subsystem
  Visualize hom transf5 : Subsystem
  Visualize hom transf6 : Subsystem
  Visualize hom transf7 : Subsystem
  Visualize hom transf8 : Subsystem
  "inertial -> rpy" : Selector  InputPortWidth=12  IndexOptions=Index vector (dialog)  Indices=[1 2 3]  OutputSizes=1
  l_sole_H_root_link2 : Subsystem  mask{link_name='l_sole'}
  l_sole_H_root_link3 : Subsystem  mask{link_name='r_sole'}
  rpy : Scope
      settings: ShowLegends=on  YMin=-67.23721  YMax=159.06533
  w_H_root_link1 : Subsystem  mask{link_name='r_sole'}
      mask prompts: link_name "link name"
      mask help:
      | This block evaluates the homogeneous transformation between the world and the root link, i.e. ^wH_b. It assumes that the link specified by the variable 'link_name' has a constant position
      | w.r.t. an inertial frame, but it can rotate arbitrarily. This rotation is retrived from the IMU sensor.
      mask Display:
      | str = strrep(link_name, '_','\_');
      | port_label('output',1,['{}^{',str '}H_{root}'],'texmode','on')
      | clear str;
      | 
      | port_label('input',1,'q_j','texmode','on')
      | 
      | port_label('input',2,'inertial','texmode','on')
  w_H_root_link4 : Subsystem  mask{link_name='l_sole'}
      mask prompts: link_name "link name"
      mask help:
      | This block evaluates the homogeneous transformation between the world and the root link, i.e. ^wH_b. It assumes that the link specified by the variable 'link_name' has a constant position
      | w.r.t. an inertial frame, but it can rotate arbitrarily. This rotation is retrived from the IMU sensor.
      mask Display:
      | str = strrep(link_name, '_','\_');
      | port_label('output',1,['{}^{',str '}H_{root}'],'texmode','on')
      | clear str;
      | 
      | port_label('input',1,'q_j','texmode','on')
      | 
      | port_label('input',2,'inertial','texmode','on')
  wires:
  inertial/1 -> "inertial -> rpy"/1, w_H_root_link1/2(inertial), w_H_root_link4/2(inertial)
  jointAngles/1 -> w_H_root_link4/1(qj), w_H_root_link1/1(qj), l_sole_H_root_link3/1(qj), l_sole_H_root_link2/1(qj)
  l_sole_H_root_link2/1(link_name_H_root_link) -> Visualize hom transf6/1(H), Inv\*/1  "l_sole_H_root_link"
  Inv\*/1 -> Visualize hom transf7/1(H)
  w_H_root_link4/1(w_H_root) -> Inv\*/2, Visualize hom transf8/1(H)
  "inertial -> rpy"/1 -> rpy/1
  l_sole_H_root_link3/1(link_name_H_root_link) -> Inv\*1/1, Visualize hom transf2/1(H)  "r_sole_H_root_link"
  Inv\*1/1 -> Visualize hom transf4/1(H)
  w_H_root_link1/1(w_H_root) -> Visualize hom transf5/1(H), Inv\*1/2

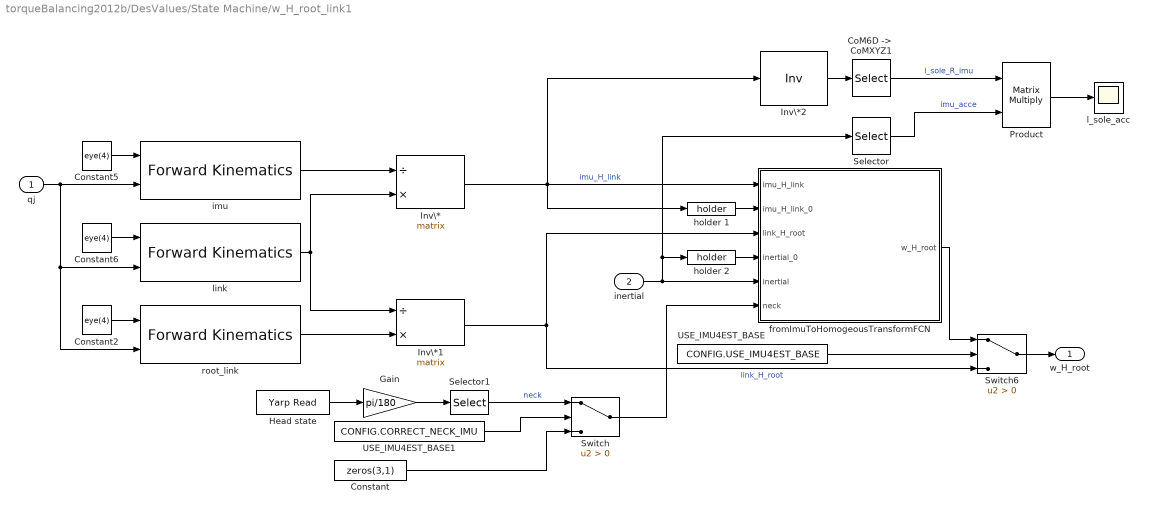
== system torqueBalancing2012b/DesValues/State Machine/w_H_root_link1 ==
  qj : Inport
  inertial : Inport  Port=2
  "CoM6D ->  CoMXYZ1" : Selector  NumberOfDimensions=2  InputPortWidth=7  IndexOptions=Index vector (dialog),Index vector (dialog)  Indices=[1 2 3],[1 2 3]  OutputSizes=1,1
  Constant : Constant  Value=zeros(3,1)
  Constant2 : Constant  Value=eye(4)
  Constant5 : Constant  Value=eye(4)
  Constant6 : Constant  Value=eye(4)
  Gain : Gain  Gain=pi/180
  Head state : WBToolboxLibrary/Utilities/Yarp Read  portName=[WBT_robotName, '/head/state:o']  signalSize=6  blocking=off  timestamp=off  autoconnect=on  errorOnConnection=off
  Inv\* : Product  Inputs=/*  Multiplication=Matrix(*)
  Inv\*1 : Product  Inputs=/*  Multiplication=Matrix(*)
  Inv\*2 : Product  Inputs=/  Multiplication=Matrix(*)
  Product : Product  Multiplication=Matrix(*)
  Selector : Selector  InputPortWidth=12  IndexOptions=Index vector (dialog)  Indices=[4 5 6 ]  OutputSizes=1
  Selector1 : Selector  InputPortWidth=6  IndexOptions=Index vector (dialog)  Indices=[1:3]  OutputSizes=1
  Switch : Switch  Criteria=u2 > Threshold
  Switch6 : Switch  Criteria=u2 > Threshold
  USE_IMU4EST_BASE : Constant  Value=CONFIG.USE_IMU4EST_BASE
  USE_IMU4EST_BASE1 : Constant  Value=CONFIG.CORRECT_NECK_IMU
  fromImuToHomogeousTransformFCN : MATLAB Function  TreatAsAtomicUnit=on
  holder 1 : WBToolboxLibrary/Utilities/holder 
  holder 2 : WBToolboxLibrary/Utilities/holder 
  imu : WBToolboxLibrary/wholeBodyModel/Kinematics/Forward Kinematics  frameName='imu_frame'  robotName=WBT_robotName  localName=WBT_modelName  wbiFile=WBT_wbiFilename  wbiList=WBT_wbiList
  l_sole_acc : Scope
      settings: ShowLegends=on  TimeRange=60  YMin=-4.47309  YMax=14.2668
  link : WBToolboxLibrary/wholeBodyModel/Kinematics/Forward Kinematics  frameName=link_name  robotName=WBT_robotName  localName=WBT_modelName  wbiFile=WBT_wbiFilename  wbiList=WBT_wbiList
  root_link : WBToolboxLibrary/wholeBodyModel/Kinematics/Forward Kinematics  frameName='root_link'  robotName=WBT_robotName  localName=WBT_modelName  wbiFile=WBT_wbiFilename  wbiList=WBT_wbiList
  w_H_root : Outport
  wires:
  Constant5/1 -> imu/1
  Inv\*/1 -> Inv\*2/1, holder 1/1, fromImuToHomogeousTransformFCN/1(imu_H_link)  "imu_H_link"
  imu/1 -> Inv\*/1
  Constant6/1 -> link/1
  Inv\*1/1 -> Switch6/3, fromImuToHomogeousTransformFCN/3(link_H_root)  "link_H_root"
  link/1 -> Inv\*/2, Inv\*1/1
  inertial/1 -> Selector/1, holder 2/1, fromImuToHomogeousTransformFCN/5(inertial)
  Switch6/1 -> w_H_root/1
  USE_IMU4EST_BASE/1 -> Switch6/2
  fromImuToHomogeousTransformFCN/1(w_H_root) -> Switch6/1
  Constant2/1 -> root_link/1
  qj/1 -> root_link/2, link/2, imu/2
  root_link/1 -> Inv\*1/2
  holder 1/1 -> fromImuToHomogeousTransformFCN/2(imu_H_link_0)
  holder 2/1 -> fromImuToHomogeousTransformFCN/4(inertial_0)
  Inv\*2/1 -> "CoM6D ->  CoMXYZ1"/1
  "CoM6D ->  CoMXYZ1"/1 -> Product/1  "l_sole_R_imu"
  Selector/1 -> Product/2  "imu_acce"
  Product/1 -> l_sole_acc/1
  Head state/1 -> Gain/1
  Selector1/1 -> Switch/1  "neck"
  USE_IMU4EST_BASE1/1 -> Switch/2
  Switch/1 -> fromImuToHomogeousTransformFCN/6(neck)
  Gain/1 -> Selector1/1
  Constant/1 -> Switch/3

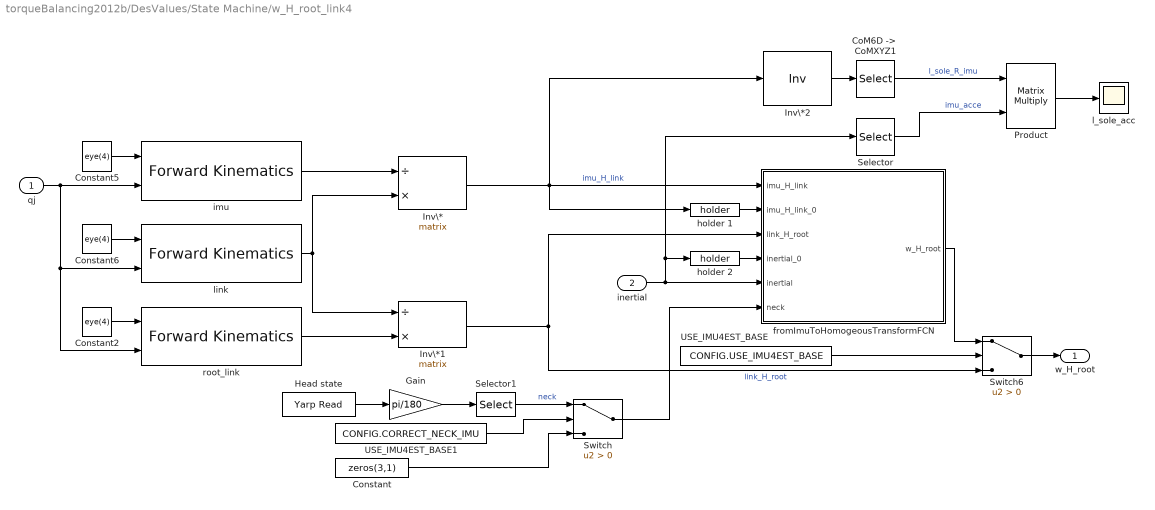
== system torqueBalancing2012b/DesValues/State Machine/w_H_root_link4 ==
  qj : Inport
  inertial : Inport  Port=2
  "CoM6D ->  CoMXYZ1" : Selector  NumberOfDimensions=2  InputPortWidth=7  IndexOptions=Index vector (dialog),Index vector (dialog)  Indices=[1 2 3],[1 2 3]  OutputSizes=1,1
  Constant : Constant  Value=zeros(3,1)
  Constant2 : Constant  Value=eye(4)
  Constant5 : Constant  Value=eye(4)
  Constant6 : Constant  Value=eye(4)
  Gain : Gain  Gain=pi/180
  Head state : WBToolboxLibrary/Utilities/Yarp Read  portName=[WBT_robotName, '/head/state:o']  signalSize=6  blocking=off  timestamp=off  autoconnect=on  errorOnConnection=off
  Inv\* : Product  Inputs=/*  Multiplication=Matrix(*)
  Inv\*1 : Product  Inputs=/*  Multiplication=Matrix(*)
  Inv\*2 : Product  Inputs=/  Multiplication=Matrix(*)
  Product : Product  Multiplication=Matrix(*)
  Selector : Selector  InputPortWidth=12  IndexOptions=Index vector (dialog)  Indices=[4 5 6 ]  OutputSizes=1
  Selector1 : Selector  InputPortWidth=6  IndexOptions=Index vector (dialog)  Indices=[1:3]  OutputSizes=1
  Switch : Switch  Criteria=u2 > Threshold
  Switch6 : Switch  Criteria=u2 > Threshold
  USE_IMU4EST_BASE : Constant  Value=CONFIG.USE_IMU4EST_BASE
  USE_IMU4EST_BASE1 : Constant  Value=CONFIG.CORRECT_NECK_IMU
  fromImuToHomogeousTransformFCN : MATLAB Function  TreatAsAtomicUnit=on
  holder 1 : WBToolboxLibrary/Utilities/holder 
  holder 2 : WBToolboxLibrary/Utilities/holder 
  imu : WBToolboxLibrary/wholeBodyModel/Kinematics/Forward Kinematics  frameName='imu_frame'  robotName=WBT_robotName  localName=WBT_modelName  wbiFile=WBT_wbiFilename  wbiList=WBT_wbiList
  l_sole_acc : Scope
      settings: ShowLegends=on  TimeRange=60  YMin=-4.47309  YMax=14.2668
  link : WBToolboxLibrary/wholeBodyModel/Kinematics/Forward Kinematics  frameName=link_name  robotName=WBT_robotName  localName=WBT_modelName  wbiFile=WBT_wbiFilename  wbiList=WBT_wbiList
  root_link : WBToolboxLibrary/wholeBodyModel/Kinematics/Forward Kinematics  frameName='root_link'  robotName=WBT_robotName  localName=WBT_modelName  wbiFile=WBT_wbiFilename  wbiList=WBT_wbiList
  w_H_root : Outport
  wires:
  Constant5/1 -> imu/1
  Inv\*/1 -> Inv\*2/1, holder 1/1, fromImuToHomogeousTransformFCN/1(imu_H_link)  "imu_H_link"
  imu/1 -> Inv\*/1
  Constant6/1 -> link/1
  Inv\*1/1 -> Switch6/3, fromImuToHomogeousTransformFCN/3(link_H_root)  "link_H_root"
  link/1 -> Inv\*/2, Inv\*1/1
  inertial/1 -> Selector/1, holder 2/1, fromImuToHomogeousTransformFCN/5(inertial)
  Switch6/1 -> w_H_root/1
  USE_IMU4EST_BASE/1 -> Switch6/2
  fromImuToHomogeousTransformFCN/1(w_H_root) -> Switch6/1
  Constant2/1 -> root_link/1
  qj/1 -> root_link/2, link/2, imu/2
  root_link/1 -> Inv\*1/2
  holder 1/1 -> fromImuToHomogeousTransformFCN/2(imu_H_link_0)
  holder 2/1 -> fromImuToHomogeousTransformFCN/4(inertial_0)
  Inv\*2/1 -> "CoM6D ->  CoMXYZ1"/1
  "CoM6D ->  CoMXYZ1"/1 -> Product/1  "l_sole_R_imu"
  Selector/1 -> Product/2  "imu_acce"
  Product/1 -> l_sole_acc/1
  Head state/1 -> Gain/1
  Selector1/1 -> Switch/1  "neck"
  USE_IMU4EST_BASE1/1 -> Switch/2
  Switch/1 -> fromImuToHomogeousTransformFCN/6(neck)
  Gain/1 -> Selector1/1
  Constant/1 -> Switch/3

== system torqueBalancing2012b/DesValues/State Machine/xCom ==
  qj : Inport
  w_H_b : Inport  Port=2
  "CoM6D ->  CoMXYZ2" : Selector  NumberOfDimensions=2  InputPortWidth=7  IndexOptions=Index vector (dialog),Index vector (dialog)  Indices=[1 2 3],[4]  OutputSizes=1,1
  com : WBToolboxLibrary/wholeBodyModel/Kinematics/Forward Kinematics  frameName='com'  robotName=WBT_robotName  localName=WBT_modelName  wbiFile=WBT_wbiFilename  wbiList=WBT_wbiList
  xCom : Outport
  wires:
  qj/1 -> com/2
  "CoM6D ->  CoMXYZ2"/1 -> xCom/1
  com/1 -> "CoM6D ->  CoMXYZ2"/1
  w_H_b/1 -> com/1

== system torqueBalancing2012b/DesValues/State Machine/xCom1 ==
  qj : Inport
  w_H_b : Inport  Port=2
  "CoM6D ->  CoMXYZ2" : Selector  NumberOfDimensions=2  InputPortWidth=7  IndexOptions=Index vector (dialog),Index vector (dialog)  Indices=[1 2 3],[4]  OutputSizes=1,1
  com : WBToolboxLibrary/wholeBodyModel/Kinematics/Forward Kinematics  frameName='com'  robotName=WBT_robotName  localName=WBT_modelName  wbiFile=WBT_wbiFilename  wbiList=WBT_wbiList
  xCom : Outport
  wires:
  qj/1 -> com/2
  "CoM6D ->  CoMXYZ2"/1 -> xCom/1
  com/1 -> "CoM6D ->  CoMXYZ2"/1
  w_H_b/1 -> com/1

== system torqueBalancing2012b/DesValues/State Machine StandUp/Visualise extrnal wrenches   ==
  wL_arm : Inport
  wR_arm : Inport  Port=2
  wL_WBDT : Inport  Port=3
  wR_WBDT : Inport  Port=4
  state : Inport  Port=5
  Enable : EnablePort
  MATLAB Function : MATLAB Function  TreatAsAtomicUnit=on
  MATLAB Function1 : MATLAB Function  TreatAsAtomicUnit=on
  Sum : Sum  Inputs=++|
  Sum1 : Sum  Inputs=++|
  left arm ext wrench : Scope  NumInputPorts=3
      settings: ShowLegends=on  YMin=-15.54616~-12.5~0.5  YMax=18.57872~12.5~5.5  SaveName=ScopeData2
  left foot ext wrench : Scope  NumInputPorts=3
      settings: ShowLegends=on  YMin=-36.27271~-17.5~0.625  YMax=205.93985~157.5~4.375
  right arm ext wrench : Scope  NumInputPorts=3
      settings: ShowLegends=on  YMin=-8.37727~-1.25~0.625  YMax=31.31102~11.25~4.375
  right foot ext wrench : Scope  NumInputPorts=3
      settings: ShowLegends=on  TimeRange=42.68  YMin=-37.58616~-17.5~0.625  YMax=186.20333~157.5~4.375  SaveName=ScopeData2
  sum foot ext wrench : Scope  NumInputPorts=3
      settings: ShowLegends=on  TimeRange=42.68  YMin=71.63562~220.01645~0.625  YMax=144.29782~306.36513~4.375  SaveName=ScopeData3
  wires:
  wR_WBDT/1 -> Sum/2, right foot ext wrench/1  "wR_WBDT"
  wL_WBDT/1 -> Sum/1, left foot ext wrench/1  "wL_WBDT"
  MATLAB Function/1(thresholdContactLeft) -> left foot ext wrench/2, Sum1/1  "thresholdContactLeft"
  MATLAB Function/2(thresholdContactRight) -> Sum1/2, right foot ext wrench/2  "thresholdContactRight"
  MATLAB Function1/2(thresholdArmContactRight) -> right arm ext wrench/2
  MATLAB Function1/1(thresholdArmContactLeft) -> left arm ext wrench/2
  wR_arm/1 -> right arm ext wrench/1
  wL_arm/1 -> left arm ext wrench/1
  state/1 -> MATLAB Function1/1(state), right foot ext wrench/3, left foot ext wrench/3, right arm ext wrench/3, left arm ext wrench/3, MATLAB Function/1(state), sum foot ext wrench/3
  Sum/1 -> sum foot ext wrench/1
  Sum1/1 -> sum foot ext wrench/2

== system torqueBalancing2012b/DesValues/State Machine StandUp/nu ==
  qj : Inport
  w_H_b : Inport  Port=2
  "constraints " : Inport  Port=3
  Get Estimate : WBToolboxLibrary/wholeBodyStates/Get Estimate  estimateType=Joints Velocity  robotName=WBT_robotName  localName=WBT_modelName  wbiFile=WBT_wbiFilename  wbiList=WBT_wbiList
  Jacobian l_sole : WBToolboxLibrary/wholeBodyModel/Jacobians/Jacobian  frameName='l_sole'  robotName=WBT_robotName  localName=WBT_modelName  wbiFile=WBT_wbiFilename  wbiList=WBT_wbiList
  Jacobian r_sole : WBToolboxLibrary/wholeBodyModel/Jacobians/Jacobian  frameName='r_sole'  robotName=WBT_robotName  localName=WBT_modelName  wbiFile=WBT_wbiFilename  wbiList=WBT_wbiList
  MATLAB Function : MATLAB Function  TreatAsAtomicUnit=on
  Mux : Mux  Inputs=2
  vb + Dqj : Outport
  wires:
  Get Estimate/1 -> MATLAB Function/4(qD), Mux/2
  Mux/1 -> vb + Dqj/1
  Jacobian r_sole/1 -> MATLAB Function/2(JcRightFoot)
  "constraints "/1 -> MATLAB Function/3(activeFeetConstraints)
  MATLAB Function/1(y) -> Mux/1
  Jacobian l_sole/1 -> MATLAB Function/1(JcLeftFoot)
  qj/1 -> Jacobian r_sole/2, Jacobian l_sole/2
  w_H_b/1 -> Jacobian r_sole/1, Jacobian l_sole/1

== system torqueBalancing2012b/DesValues/State Machine StandUp/visualise inertial ==
  jointAngles : Inport
  inertial : Inport  Port=2
  Enable : EnablePort
  Inv\* : Product  Inputs=/*  Multiplication=Matrix(*)
  Inv\*1 : Product  Inputs=/*  Multiplication=Matrix(*)
  Visualize hom transf2 : Subsystem
  Visualize hom transf4 : Subsystem
  Visualize hom transf5 : Subsystem
  Visualize hom transf6 : Subsystem
  Visualize hom transf7 : Subsystem
  Visualize hom transf8 : Subsystem
  "inertial -> rpy" : Selector  InputPortWidth=12  IndexOptions=Index vector (dialog)  Indices=[1 2 3]  OutputSizes=1
  l_sole_H_root_link2 : Subsystem  mask{link_name='l_sole'}
  l_sole_H_root_link3 : Subsystem  mask{link_name='r_sole'}
  rpy : Scope
      settings: ShowLegends=on  YMin=-67.23721  YMax=159.06533
  w_H_root_link1 : Subsystem  mask{link_name='r_sole'}
      mask prompts: link_name "link name"
      mask help:
      | This block evaluates the homogeneous transformation between the world and the root link, i.e. ^wH_b. It assumes that the link specified by the variable 'link_name' has a constant position
      | w.r.t. an inertial frame, but it can rotate arbitrarily. This rotation is retrived from the IMU sensor.
      mask Display:
      | str = strrep(link_name, '_','\_');
      | port_label('output',1,['{}^{',str '}H_{root}'],'texmode','on')
      | clear str;
      | 
      | port_label('input',1,'q_j','texmode','on')
      | 
      | port_label('input',2,'inertial','texmode','on')
  w_H_root_link4 : Subsystem  mask{link_name='l_sole'}
      mask prompts: link_name "link name"
      mask help:
      | This block evaluates the homogeneous transformation between the world and the root link, i.e. ^wH_b. It assumes that the link specified by the variable 'link_name' has a constant position
      | w.r.t. an inertial frame, but it can rotate arbitrarily. This rotation is retrived from the IMU sensor.
      mask Display:
      | str = strrep(link_name, '_','\_');
      | port_label('output',1,['{}^{',str '}H_{root}'],'texmode','on')
      | clear str;
      | 
      | port_label('input',1,'q_j','texmode','on')
      | 
      | port_label('input',2,'inertial','texmode','on')
  wires:
  inertial/1 -> "inertial -> rpy"/1, w_H_root_link1/2(inertial), w_H_root_link4/2(inertial)
  jointAngles/1 -> w_H_root_link4/1(qj), w_H_root_link1/1(qj), l_sole_H_root_link3/1(qj), l_sole_H_root_link2/1(qj)
  l_sole_H_root_link2/1(link_name_H_root_link) -> Visualize hom transf6/1(H), Inv\*/1  "l_sole_H_root_link"
  Inv\*/1 -> Visualize hom transf7/1(H)
  w_H_root_link4/1(w_H_root) -> Inv\*/2, Visualize hom transf8/1(H)
  "inertial -> rpy"/1 -> rpy/1
  l_sole_H_root_link3/1(link_name_H_root_link) -> Inv\*1/1, Visualize hom transf2/1(H)  "r_sole_H_root_link"
  Inv\*1/1 -> Visualize hom transf4/1(H)
  w_H_root_link1/1(w_H_root) -> Visualize hom transf5/1(H), Inv\*1/2
